simulink model "IEEE33bus_SmartInverter_Hybrid_PSO_English"  (R2026a)
settings: Solver=VariableStepAuto
PreLoadFcn:
  | try, if exist('startup_project','file') == 2, startup_project(); end, catch ME, disp(['PreLoadFcn warning: ' ME.message]); end
InitFcn:
  | try, if exist('ieee33_data','file') == 2, assignin('base','ieee33_visual_network',ieee33_data()); end; if exist('default_control_params','file') == 2, assignin('base','ieee33_visual_control_params',default_control_params()); end; disp('IEEE33 visualization initialized. MATLAB scripts provide numerical results.'); catch ME, disp(['InitFcn warning: ' ME.message]); end
StopFcn:
  | try, disp('IEEE33 visualization stopped. Use main_generate_final_results for refreshed tables and figures.'); catch ME, disp(['StopFcn warning: ' ME.message]); end
settings Model: Creator=ismahin  LastModifiedBy=ismahin

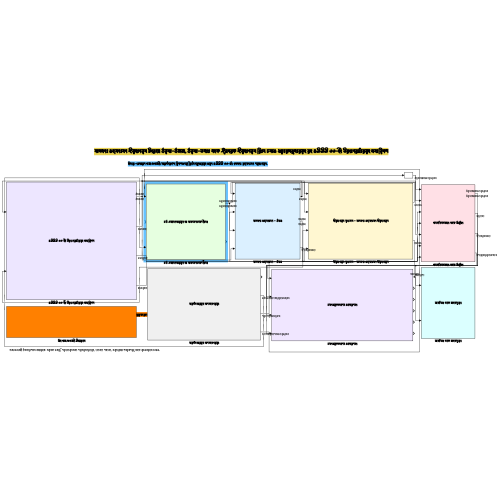
[thumbnail: Simulink's stored preview of the top-level diagram]
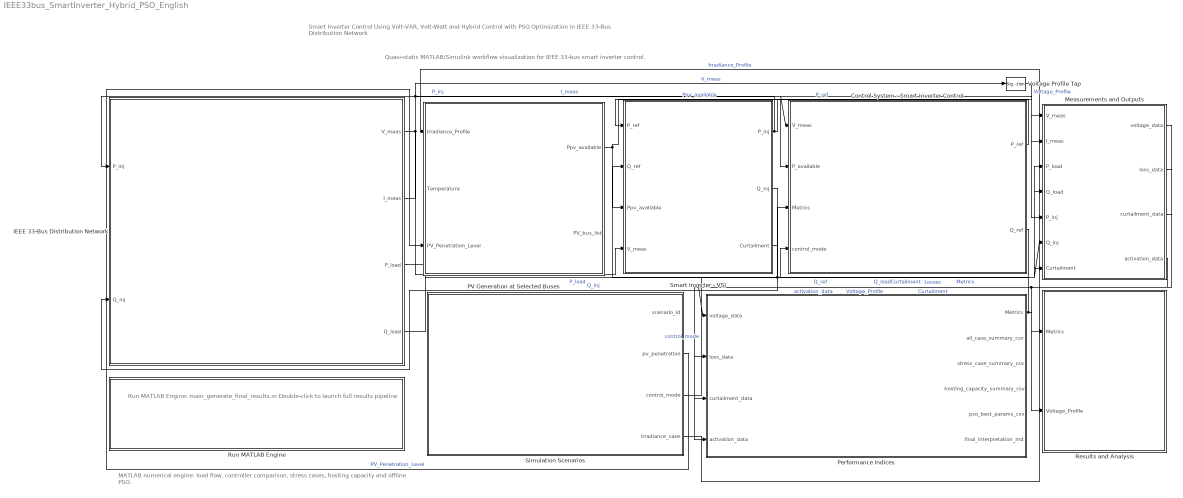
== system IEEE33bus_SmartInverter_Hybrid_PSO_English ==
  note: Run MATLAB Engine:\nmain_generate_final_results.m\nDouble-click to launch full results pipeline
  note: Smart Inverter Control Using Volt-VAR, Volt-Watt and Hybrid Control with PSO Optimization in IEEE 33-Bus Distribution Network
  note: Quasi-static MATLAB/Simulink workflow visualization for IEEE 33-bus smart inverter control.
  note: MATLAB numerical engine: load flow, controller comparison, stress cases, hosting capacity and offline PSO.
  Control System - Smart Inverter Control : Subsystem
      mask Display: color('black'); patch([0 1 1 0],[0 0 1 1],[1.000 0.970 0.820]); disp('Control System - Smart Inverter Control');
  IEEE 33-Bus Distribution Network : Subsystem
      mask Display: color('black'); patch([0 1 1 0],[0 0 1 1],[0.930 0.900 1.000]); disp('IEEE 33-Bus Distribution Network');
  Measurements and Outputs : Subsystem
      mask Display: color('black'); patch([0 1 1 0],[0 0 1 1],[1.000 0.880 0.900]); disp('Measurements and Outputs');
  PV Generation at Selected Buses : Subsystem
      mask Display: color('black'); patch([0 1 1 0],[0 0 1 1],[0.900 1.000 0.880]); disp('PV Generation at Selected Buses');
  Performance Indices : Subsystem
      mask Display: color('black'); patch([0 1 1 0],[0 0 1 1],[0.940 0.900 1.000]); disp('Performance Indices');
  Results and Analysis : Subsystem
      mask Display: color('black'); patch([0 1 1 0],[0 0 1 1],[0.860 1.000 1.000]); disp('Results and Analysis');
  Run MATLAB Engine : Subsystem
      settings: OpenFcn=try, evalin('base','main_generate_final_results'); catch ME, disp(['Pipeline launch failed: ' ME.message]); end
  Simulation Scenarios : Subsystem
      mask Display: color('black'); patch([0 1 1 0],[0 0 1 1],[0.940 0.940 0.940]); disp('Simulation Scenarios');
  Smart Inverter - VSI : Subsystem
      mask Display: color('black'); patch([0 1 1 0],[0 0 1 1],[0.860 0.940 1.000]); disp('Smart Inverter - VSI');
  Voltage Profile Tap : SignalSpecification
  wires:
  Simulation Scenarios/4(irradiance_case) -> PV Generation at Selected Buses/1(Irradiance_Profile)  "Irradiance_Profile"
  Simulation Scenarios/2(pv_penetration) -> PV Generation at Selected Buses/3(PV_Penetration_Level)  "PV_Penetration_Level"
  Simulation Scenarios/3(control_mode) -> Control System - Smart Inverter Control/4(control_mode)  "control_mode"
  PV Generation at Selected Buses/1(Ppv_available) -> Smart Inverter - VSI/3(Ppv_available), Control System - Smart Inverter Control/2(P_available)  "Ppv_available"
  IEEE 33-Bus Distribution Network/1(V_meas) -> Control System - Smart Inverter Control/1(V_meas), Voltage Profile Tap/1, Smart Inverter - VSI/4(V_meas)  "V_meas"
  Control System - Smart Inverter Control/1(P_ref) -> Smart Inverter - VSI/1(P_ref)  "P_ref"
  Control System - Smart Inverter Control/2(Q_ref) -> Smart Inverter - VSI/2(Q_ref)  "Q_ref"
  Smart Inverter - VSI/1(P_inj) -> IEEE 33-Bus Distribution Network/1(P_inj), Measurements and Outputs/5(P_inj)  "P_inj"
  Smart Inverter - VSI/2(Q_inj) -> IEEE 33-Bus Distribution Network/2(Q_inj), Measurements and Outputs/6(Q_inj)  "Q_inj"
  Voltage Profile Tap/1 -> Measurements and Outputs/1(V_meas)  "Voltage_Profile"
  IEEE 33-Bus Distribution Network/2(I_meas) -> Measurements and Outputs/2(I_meas)  "I_meas"
  IEEE 33-Bus Distribution Network/3(P_load) -> Measurements and Outputs/3(P_load)  "P_load"
  IEEE 33-Bus Distribution Network/4(Q_load) -> Measurements and Outputs/4(Q_load)  "Q_load"
  Smart Inverter - VSI/3(Curtailment) -> Measurements and Outputs/7(Curtailment)  "Curtailment"
  Measurements and Outputs/1(voltage_data) -> Performance Indices/1(voltage_data), Results and Analysis/2(Voltage_Profile)  "Voltage_Profile"
  Measurements and Outputs/2(loss_data) -> Performance Indices/2(loss_data)  "Losses"
  Measurements and Outputs/3(curtailment_data) -> Performance Indices/3(curtailment_data)  "Curtailment"
  Measurements and Outputs/4(activation_data) -> Performance Indices/4(activation_data)  "activation_data"
  Performance Indices/1(Metrics) -> Results and Analysis/1(Metrics), Control System - Smart Inverter Control/3(Metrics)  "Metrics"

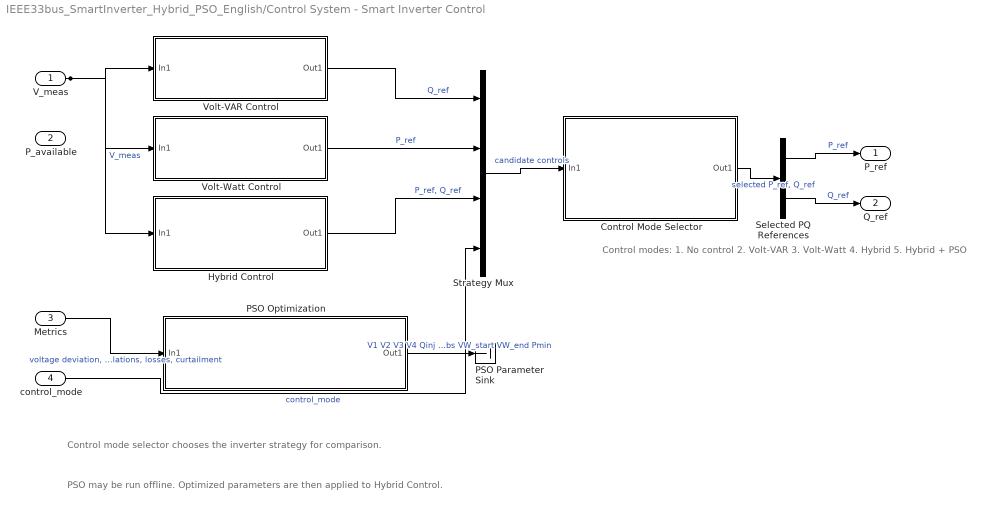
== system IEEE33bus_SmartInverter_Hybrid_PSO_English/Control System - Smart Inverter Control ==
  note: Control modes:\n1. No control\n2. Volt-VAR\n3. Volt-Watt\n4. Hybrid\n5. Hybrid + PSO
  note: Control mode selector chooses the inverter strategy for comparison.
  note: PSO may be run offline. Optimized parameters are then applied to Hybrid Control.
  V_meas : Inport
  P_available : Inport  Port=2
  Metrics : Inport  Port=3
  control_mode : Inport  Port=4
  Control Mode Selector : Subsystem
      mask Display: color('black'); patch([0 1 1 0],[0 0 1 1],[1.000 0.950 0.780]); disp('Control Mode Selector');
  Hybrid Control : Subsystem
      mask Display: color('black'); patch([0 1 1 0],[0 0 1 1],[1.000 0.900 0.580]); disp('Hybrid: Volt-VAR + Volt-Watt');
  PSO Optimization : Subsystem
      mask Display: color('black'); patch([0 1 1 0],[0 0 1 1],[1.000 0.780 0.900]); disp('PSO Optimization (Offline)');
  PSO Parameter Sink : Terminator
  Selected PQ References : Demux  Outputs=2
  Strategy Mux : Mux
  Volt-VAR Control : Subsystem
      mask Display: color('black'); patch([0 1 1 0],[0 0 1 1],[1.000 0.930 0.660]); disp('Volt-VAR Control  Q = f(V)');
  Volt-Watt Control : Subsystem
      mask Display: color('black'); patch([0 1 1 0],[0 0 1 1],[1.000 0.930 0.660]); disp('Volt-Watt Control  P = f(V)');
  P_ref : Outport
  Q_ref : Outport  Port=2
  wires:
  V_meas/1 -> Volt-VAR Control/1(In1), Volt-Watt Control/1(In1), Hybrid Control/1(In1)  "V_meas"
  Metrics/1 -> PSO Optimization/1(In1)  "voltage deviation, violations, losses, curtailment"
  Volt-VAR Control/1(Out1) -> Strategy Mux/1  "Q_ref"
  Volt-Watt Control/1(Out1) -> Strategy Mux/2  "P_ref"
  Hybrid Control/1(Out1) -> Strategy Mux/3  "P_ref, Q_ref"
  control_mode/1 -> Strategy Mux/4  "control_mode"
  Strategy Mux/1 -> Control Mode Selector/1(In1)  "candidate controls"
  Control Mode Selector/1(Out1) -> Selected PQ References/1  "selected P_ref, Q_ref"
  Selected PQ References/1 -> P_ref/1  "P_ref"
  Selected PQ References/2 -> Q_ref/1  "Q_ref"
  PSO Optimization/1(Out1) -> PSO Parameter Sink/1  "V1 V2 V3 V4 Qinj Qabs VW_start VW_end Pmin"

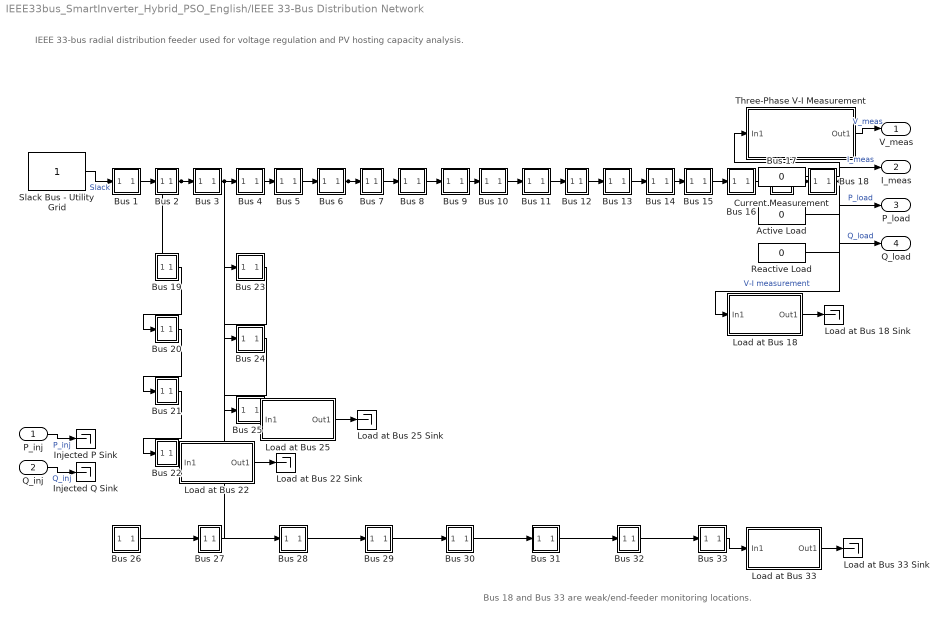
== system IEEE33bus_SmartInverter_Hybrid_PSO_English/IEEE 33-Bus Distribution Network ==
  note: IEEE 33-bus radial distribution feeder used for voltage regulation and PV hosting capacity analysis.
  note: Bus 18 and Bus 33 are weak/end-feeder monitoring locations.
  P_inj : Inport
  Q_inj : Inport  Port=2
  Active Load : Constant  Value=0
  Bus 1 : Subsystem
      mask Display: color('black'); patch([0 1 1 0],[0 0 1 1],[0.820 0.820 0.820]); disp('1');
  Bus 10 : Subsystem
      mask Display: color('black'); patch([0 1 1 0],[0 0 1 1],[0.820 0.820 0.820]); disp('10');
  Bus 11 : Subsystem
      mask Display: color('black'); patch([0 1 1 0],[0 0 1 1],[0.820 0.820 0.820]); disp('11');
  Bus 12 : Subsystem
      mask Display: color('black'); patch([0 1 1 0],[0 0 1 1],[0.820 0.820 0.820]); disp('12');
  Bus 13 : Subsystem
      mask Display: color('black'); patch([0 1 1 0],[0 0 1 1],[0.820 0.820 0.820]); disp('13');
  Bus 14 : Subsystem
      mask Display: color('black'); patch([0 1 1 0],[0 0 1 1],[0.820 0.820 0.820]); disp('14');
  Bus 15 : Subsystem
      mask Display: color('black'); patch([0 1 1 0],[0 0 1 1],[0.820 0.820 0.820]); disp('15');
  Bus 16 : Subsystem
      mask Display: color('black'); patch([0 1 1 0],[0 0 1 1],[0.820 0.820 0.820]); disp('16');
  Bus 17 : Subsystem
      mask Display: color('black'); patch([0 1 1 0],[0 0 1 1],[0.820 0.820 0.820]); disp('17');
  Bus 18 : Subsystem
      mask Display: color('black'); patch([0 1 1 0],[0 0 1 1],[0.820 0.820 0.820]); disp('18');
  Bus 19 : Subsystem
      mask Display: color('black'); patch([0 1 1 0],[0 0 1 1],[0.820 0.820 0.820]); disp('19');
  Bus 2 : Subsystem
      mask Display: color('black'); patch([0 1 1 0],[0 0 1 1],[0.820 0.820 0.820]); disp('2');
  Bus 20 : Subsystem
      mask Display: color('black'); patch([0 1 1 0],[0 0 1 1],[0.820 0.820 0.820]); disp('20');
  Bus 21 : Subsystem
      mask Display: color('black'); patch([0 1 1 0],[0 0 1 1],[0.820 0.820 0.820]); disp('21');
  Bus 22 : Subsystem
      mask Display: color('black'); patch([0 1 1 0],[0 0 1 1],[0.820 0.820 0.820]); disp('22');
  Bus 23 : Subsystem
      mask Display: color('black'); patch([0 1 1 0],[0 0 1 1],[0.820 0.820 0.820]); disp('23');
  Bus 24 : Subsystem
      mask Display: color('black'); patch([0 1 1 0],[0 0 1 1],[0.820 0.820 0.820]); disp('24');
  Bus 25 : Subsystem
      mask Display: color('black'); patch([0 1 1 0],[0 0 1 1],[0.820 0.820 0.820]); disp('25');
  Bus 26 : Subsystem
      mask Display: color('black'); patch([0 1 1 0],[0 0 1 1],[0.820 0.820 0.820]); disp('26');
  Bus 27 : Subsystem
      mask Display: color('black'); patch([0 1 1 0],[0 0 1 1],[0.820 0.820 0.820]); disp('27');
  Bus 28 : Subsystem
      mask Display: color('black'); patch([0 1 1 0],[0 0 1 1],[0.820 0.820 0.820]); disp('28');
  Bus 29 : Subsystem
      mask Display: color('black'); patch([0 1 1 0],[0 0 1 1],[0.820 0.820 0.820]); disp('29');
  Bus 3 : Subsystem
      mask Display: color('black'); patch([0 1 1 0],[0 0 1 1],[0.820 0.820 0.820]); disp('3');
  Bus 30 : Subsystem
      mask Display: color('black'); patch([0 1 1 0],[0 0 1 1],[0.820 0.820 0.820]); disp('30');
  Bus 31 : Subsystem
      mask Display: color('black'); patch([0 1 1 0],[0 0 1 1],[0.820 0.820 0.820]); disp('31');
  Bus 32 : Subsystem
      mask Display: color('black'); patch([0 1 1 0],[0 0 1 1],[0.820 0.820 0.820]); disp('32');
  Bus 33 : Subsystem
      mask Display: color('black'); patch([0 1 1 0],[0 0 1 1],[0.820 0.820 0.820]); disp('33');
  Bus 4 : Subsystem
      mask Display: color('black'); patch([0 1 1 0],[0 0 1 1],[0.820 0.820 0.820]); disp('4');
  Bus 5 : Subsystem
      mask Display: color('black'); patch([0 1 1 0],[0 0 1 1],[0.820 0.820 0.820]); disp('5');
  Bus 6 : Subsystem
      mask Display: color('black'); patch([0 1 1 0],[0 0 1 1],[0.820 0.820 0.820]); disp('6');
  Bus 7 : Subsystem
      mask Display: color('black'); patch([0 1 1 0],[0 0 1 1],[0.820 0.820 0.820]); disp('7');
  Bus 8 : Subsystem
      mask Display: color('black'); patch([0 1 1 0],[0 0 1 1],[0.820 0.820 0.820]); disp('8');
  Bus 9 : Subsystem
      mask Display: color('black'); patch([0 1 1 0],[0 0 1 1],[0.820 0.820 0.820]); disp('9');
  Current Measurement : Constant  Value=0
  Injected P Sink : Terminator
  Injected Q Sink : Terminator
  Load at Bus 18 : Subsystem
      mask Display: color('black'); patch([0 1 1 0],[0 0 1 1],[1.000 0.880 0.820]); disp('Load\nBus 18');
  Load at Bus 18 Sink : Terminator
  Load at Bus 22 : Subsystem
      mask Display: color('black'); patch([0 1 1 0],[0 0 1 1],[1.000 0.880 0.820]); disp('Load\nBus 22');
  Load at Bus 22 Sink : Terminator
  Load at Bus 25 : Subsystem
      mask Display: color('black'); patch([0 1 1 0],[0 0 1 1],[1.000 0.880 0.820]); disp('Load\nBus 25');
  Load at Bus 25 Sink : Terminator
  Load at Bus 33 : Subsystem
      mask Display: color('black'); patch([0 1 1 0],[0 0 1 1],[1.000 0.880 0.820]); disp('Load\nBus 33');
  Load at Bus 33 Sink : Terminator
  Reactive Load : Constant  Value=0
  Slack Bus - Utility Grid : Constant
  Three-Phase V-I Measurement : Subsystem
      mask Display: color('black'); patch([0 1 1 0],[0 0 1 1],[1.000 0.940 0.800]); disp('Three-Phase V-I Measurement');
  V_meas : Outport
  I_meas : Outport  Port=2
  P_load : Outport  Port=3
  Q_load : Outport  Port=4
  wires:
  Slack Bus - Utility Grid/1 -> Bus 1/1(In1)  "Slack"
  Bus 1/1(Out1) -> Bus 2/1(In1)
  Bus 2/1(Out1) -> Bus 3/1(In1), Bus 19/1(In1)
  Bus 3/1(Out1) -> Bus 4/1(In1), Bus 23/1(In1)
  Bus 4/1(Out1) -> Bus 5/1(In1)
  Bus 5/1(Out1) -> Bus 6/1(In1)
  Bus 6/1(Out1) -> Bus 7/1(In1), Bus 26/1(In1)
  Bus 7/1(Out1) -> Bus 8/1(In1)
  Bus 8/1(Out1) -> Bus 9/1(In1)
  Bus 9/1(Out1) -> Bus 10/1(In1)
  Bus 10/1(Out1) -> Bus 11/1(In1)
  Bus 11/1(Out1) -> Bus 12/1(In1)
  Bus 12/1(Out1) -> Bus 13/1(In1)
  Bus 13/1(Out1) -> Bus 14/1(In1)
  Bus 14/1(Out1) -> Bus 15/1(In1)
  Bus 15/1(Out1) -> Bus 16/1(In1)
  Bus 16/1(Out1) -> Bus 17/1(In1)
  Bus 17/1(Out1) -> Bus 18/1(In1)
  Bus 19/1(Out1) -> Bus 20/1(In1)
  Bus 20/1(Out1) -> Bus 21/1(In1)
  Bus 21/1(Out1) -> Bus 22/1(In1)
  Bus 23/1(Out1) -> Bus 24/1(In1)
  Bus 24/1(Out1) -> Bus 25/1(In1)
  Bus 26/1(Out1) -> Bus 27/1(In1)
  Bus 27/1(Out1) -> Bus 28/1(In1)
  Bus 28/1(Out1) -> Bus 29/1(In1)
  Bus 29/1(Out1) -> Bus 30/1(In1)
  Bus 30/1(Out1) -> Bus 31/1(In1)
  Bus 31/1(Out1) -> Bus 32/1(In1)
  Bus 32/1(Out1) -> Bus 33/1(In1)
  Bus 18/1(Out1) -> Three-Phase V-I Measurement/1(In1), Load at Bus 18/1(In1)  "V-I measurement"
  Three-Phase V-I Measurement/1(Out1) -> V_meas/1  "V_meas"
  Current Measurement/1 -> I_meas/1  "I_meas"
  Active Load/1 -> P_load/1  "P_load"
  Reactive Load/1 -> Q_load/1  "Q_load"
  Load at Bus 18/1(Out1) -> Load at Bus 18 Sink/1
  Bus 22/1(Out1) -> Load at Bus 22/1(In1)
  Load at Bus 22/1(Out1) -> Load at Bus 22 Sink/1
  Bus 25/1(Out1) -> Load at Bus 25/1(In1)
  Load at Bus 25/1(Out1) -> Load at Bus 25 Sink/1
  Bus 33/1(Out1) -> Load at Bus 33/1(In1)
  Load at Bus 33/1(Out1) -> Load at Bus 33 Sink/1
  P_inj/1 -> Injected P Sink/1  "P_inj"
  Q_inj/1 -> Injected Q Sink/1  "Q_inj"

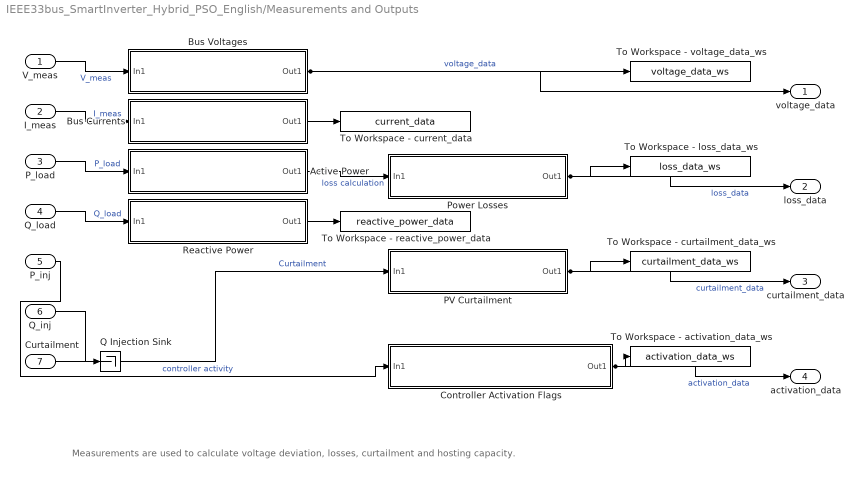
== system IEEE33bus_SmartInverter_Hybrid_PSO_English/Measurements and Outputs ==
  note: Measurements are used to calculate voltage deviation, losses, curtailment and hosting capacity.
  V_meas : Inport
  I_meas : Inport  Port=2
  P_load : Inport  Port=3
  Q_load : Inport  Port=4
  P_inj : Inport  Port=5
  Q_inj : Inport  Port=6
  Curtailment : Inport  Port=7
  Active Power : Subsystem
      mask Display: color('black'); patch([0 1 1 0],[0 0 1 1],[1.000 0.920 0.920]); disp('Active Power (kW)');
  Bus Currents : Subsystem
      mask Display: color('black'); patch([0 1 1 0],[0 0 1 1],[1.000 0.920 0.920]); disp('Bus Currents (A)');
  Bus Voltages : Subsystem
      mask Display: color('black'); patch([0 1 1 0],[0 0 1 1],[1.000 0.920 0.920]); disp('Bus Voltages (p.u.)');
  Controller Activation Flags : Subsystem
      mask Display: color('black'); patch([0 1 1 0],[0 0 1 1],[1.000 0.860 0.880]); disp('Controller Activation Flags');
  PV Curtailment : Subsystem
      mask Display: color('black'); patch([0 1 1 0],[0 0 1 1],[1.000 0.860 0.880]); disp('PV Curtailment (kWh)');
  Power Losses : Subsystem
      mask Display: color('black'); patch([0 1 1 0],[0 0 1 1],[1.000 0.860 0.880]); disp('Power Losses (kW)');
  Q Injection Sink : Terminator
  Reactive Power : Subsystem
      mask Display: color('black'); patch([0 1 1 0],[0 0 1 1],[1.000 0.920 0.920]); disp('Reactive Power (kVAr)');
  To Workspace - activation_data_ws : ToWorkspace  VariableName=activation_data_ws  SampleTime=-1
  To Workspace - current_data : ToWorkspace  VariableName=current_data  SampleTime=-1
  To Workspace - curtailment_data_ws : ToWorkspace  VariableName=curtailment_data_ws  SampleTime=-1
  To Workspace - loss_data_ws : ToWorkspace  VariableName=loss_data_ws  SampleTime=-1
  To Workspace - reactive_power_data : ToWorkspace  VariableName=reactive_power_data  SampleTime=-1
  To Workspace - voltage_data_ws : ToWorkspace  VariableName=voltage_data_ws  SampleTime=-1
  voltage_data : Outport
  loss_data : Outport  Port=2
  curtailment_data : Outport  Port=3
  activation_data : Outport  Port=4
  wires:
  V_meas/1 -> Bus Voltages/1(In1)  "V_meas"
  Bus Voltages/1(Out1) -> voltage_data/1, To Workspace - voltage_data_ws/1  "voltage_data"
  I_meas/1 -> Bus Currents/1(In1)  "I_meas"
  P_load/1 -> Active Power/1(In1)  "P_load"
  Q_load/1 -> Reactive Power/1(In1)  "Q_load"
  Active Power/1(Out1) -> Power Losses/1(In1)  "loss calculation"
  Power Losses/1(Out1) -> loss_data/1, To Workspace - loss_data_ws/1  "loss_data"
  Curtailment/1 -> PV Curtailment/1(In1)  "Curtailment"
  PV Curtailment/1(Out1) -> curtailment_data/1, To Workspace - curtailment_data_ws/1  "curtailment_data"
  P_inj/1 -> Controller Activation Flags/1(In1)  "controller activity"
  Controller Activation Flags/1(Out1) -> activation_data/1, To Workspace - activation_data_ws/1  "activation_data"
  Bus Currents/1(Out1) -> To Workspace - current_data/1
  Reactive Power/1(Out1) -> To Workspace - reactive_power_data/1
  Q_inj/1 -> Q Injection Sink/1

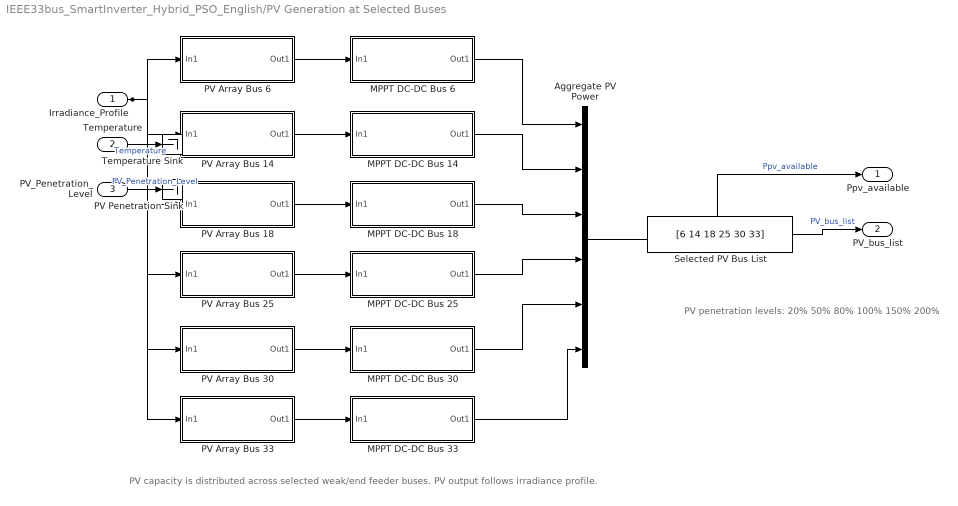
== system IEEE33bus_SmartInverter_Hybrid_PSO_English/PV Generation at Selected Buses ==
  note: PV penetration levels:\n20%\n50%\n80%\n100%\n150%\n200%
  note: PV capacity is distributed across selected weak/end feeder buses. PV output follows irradiance profile.
  Irradiance_Profile : Inport
  Temperature : Inport  Port=2
  PV_Penetration_Level : Inport  Port=3
  Aggregate PV Power : Mux  Inputs=6
  MPPT DC-DC Bus 14 : Subsystem
      mask Display: color('black'); patch([0 1 1 0],[0 0 1 1],[0.860 0.980 0.820]); disp('DC-DC / MPPT');
  MPPT DC-DC Bus 18 : Subsystem
      mask Display: color('black'); patch([0 1 1 0],[0 0 1 1],[0.860 0.980 0.820]); disp('DC-DC / MPPT');
  MPPT DC-DC Bus 25 : Subsystem
      mask Display: color('black'); patch([0 1 1 0],[0 0 1 1],[0.860 0.980 0.820]); disp('DC-DC / MPPT');
  MPPT DC-DC Bus 30 : Subsystem
      mask Display: color('black'); patch([0 1 1 0],[0 0 1 1],[0.860 0.980 0.820]); disp('DC-DC / MPPT');
  MPPT DC-DC Bus 33 : Subsystem
      mask Display: color('black'); patch([0 1 1 0],[0 0 1 1],[0.860 0.980 0.820]); disp('DC-DC / MPPT');
  MPPT DC-DC Bus 6 : Subsystem
      mask Display: color('black'); patch([0 1 1 0],[0 0 1 1],[0.860 0.980 0.820]); disp('DC-DC / MPPT');
  PV Array Bus 14 : Subsystem
      mask Display: color('black'); patch([0 1 1 0],[0 0 1 1],[0.720 0.940 0.720]); disp('PV Array\nBus 14');
  PV Array Bus 18 : Subsystem
      mask Display: color('black'); patch([0 1 1 0],[0 0 1 1],[0.720 0.940 0.720]); disp('PV Array\nBus 18');
  PV Array Bus 25 : Subsystem
      mask Display: color('black'); patch([0 1 1 0],[0 0 1 1],[0.720 0.940 0.720]); disp('PV Array\nBus 25');
  PV Array Bus 30 : Subsystem
      mask Display: color('black'); patch([0 1 1 0],[0 0 1 1],[0.720 0.940 0.720]); disp('PV Array\nBus 30');
  PV Array Bus 33 : Subsystem
      mask Display: color('black'); patch([0 1 1 0],[0 0 1 1],[0.720 0.940 0.720]); disp('PV Array\nBus 33');
  PV Array Bus 6 : Subsystem
      mask Display: color('black'); patch([0 1 1 0],[0 0 1 1],[0.720 0.940 0.720]); disp('PV Array\nBus 6');
  PV Penetration Sink : Terminator
  Selected PV Bus List : Constant  Value=[6 14 18 25 30 33]
  Temperature Sink : Terminator
  Ppv_available : Outport
  PV_bus_list : Outport  Port=2
  wires:
  Irradiance_Profile/1 -> PV Array Bus 6/1(In1), PV Array Bus 14/1(In1), PV Array Bus 18/1(In1), PV Array Bus 25/1(In1), PV Array Bus 30/1(In1), PV Array Bus 33/1(In1)
  PV Array Bus 6/1(Out1) -> MPPT DC-DC Bus 6/1(In1)
  PV Array Bus 14/1(Out1) -> MPPT DC-DC Bus 14/1(In1)
  PV Array Bus 18/1(Out1) -> MPPT DC-DC Bus 18/1(In1)
  PV Array Bus 25/1(Out1) -> MPPT DC-DC Bus 25/1(In1)
  PV Array Bus 30/1(Out1) -> MPPT DC-DC Bus 30/1(In1)
  PV Array Bus 33/1(Out1) -> MPPT DC-DC Bus 33/1(In1)
  MPPT DC-DC Bus 6/1(Out1) -> Aggregate PV Power/1
  MPPT DC-DC Bus 14/1(Out1) -> Aggregate PV Power/2
  MPPT DC-DC Bus 18/1(Out1) -> Aggregate PV Power/3
  MPPT DC-DC Bus 25/1(Out1) -> Aggregate PV Power/4
  MPPT DC-DC Bus 30/1(Out1) -> Aggregate PV Power/5
  MPPT DC-DC Bus 33/1(Out1) -> Aggregate PV Power/6
  Aggregate PV Power/1 -> Ppv_available/1  "Ppv_available"
  Selected PV Bus List/1 -> PV_bus_list/1  "PV_bus_list"
  Temperature/1 -> Temperature Sink/1  "Temperature"
  PV_Penetration_Level/1 -> PV Penetration Sink/1  "PV_Penetration_Level"

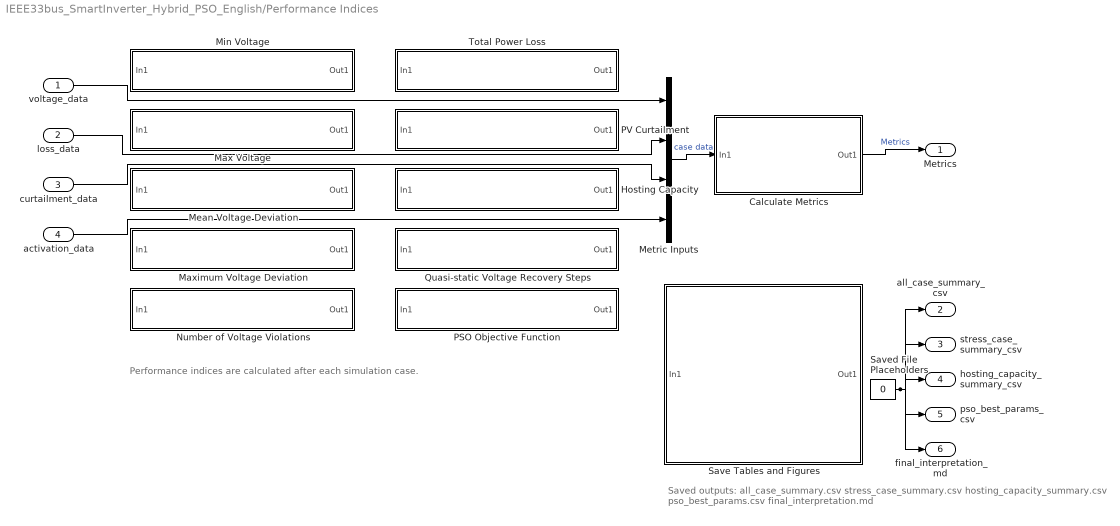
== system IEEE33bus_SmartInverter_Hybrid_PSO_English/Performance Indices ==
  note: Saved outputs:\nall_case_summary.csv\nstress_case_summary.csv\nhosting_capacity_summary.csv\npso_best_params.csv\nfinal_interpretation.md
  note: Performance indices are calculated after each simulation case.
  voltage_data : Inport
  loss_data : Inport  Port=2
  curtailment_data : Inport  Port=3
  activation_data : Inport  Port=4
  Calculate Metrics : Subsystem
      mask Display: color('black'); patch([0 1 1 0],[0 0 1 1],[0.880 0.820 1.000]); disp('Calculate Metrics');
  Hosting Capacity : Subsystem
      mask Display: color('black'); patch([0 1 1 0],[0 0 1 1],[0.960 0.930 1.000]); disp('Hosting Capacity');
  Max Voltage : Subsystem
      mask Display: color('black'); patch([0 1 1 0],[0 0 1 1],[0.960 0.930 1.000]); disp('Max Voltage');
  Maximum Voltage Deviation : Subsystem
      mask Display: color('black'); patch([0 1 1 0],[0 0 1 1],[0.960 0.930 1.000]); disp('Maximum Voltage Deviation');
  Mean Voltage Deviation : Subsystem
      mask Display: color('black'); patch([0 1 1 0],[0 0 1 1],[0.960 0.930 1.000]); disp('Mean Voltage Deviation');
  Metric Inputs : Mux
  Min Voltage : Subsystem
      mask Display: color('black'); patch([0 1 1 0],[0 0 1 1],[0.960 0.930 1.000]); disp('Min Voltage');
  Number of Voltage Violations : Subsystem
      mask Display: color('black'); patch([0 1 1 0],[0 0 1 1],[0.960 0.930 1.000]); disp('Number of Voltage Violations');
  PSO Objective Function : Subsystem
      mask Display: color('black'); patch([0 1 1 0],[0 0 1 1],[0.960 0.930 1.000]); disp('PSO Objective Function');
  PV Curtailment : Subsystem
      mask Display: color('black'); patch([0 1 1 0],[0 0 1 1],[0.960 0.930 1.000]); disp('PV Curtailment');
  Quasi-static Voltage Recovery Steps : Subsystem
      mask Display: color('black'); patch([0 1 1 0],[0 0 1 1],[0.960 0.930 1.000]); disp('Quasi-static Voltage Recovery Steps');
  Save Tables and Figures : Subsystem
      mask Display: color('black'); patch([0 1 1 0],[0 0 1 1],[0.900 0.840 1.000]); disp('Save Tables and Figures');
  Saved File Placeholders : Constant  Value=0
  Total Power Loss : Subsystem
      mask Display: color('black'); patch([0 1 1 0],[0 0 1 1],[0.960 0.930 1.000]); disp('Total Power Loss');
  Metrics : Outport
  all_case_summary_csv : Outport  Port=2
  stress_case_summary_csv : Outport  Port=3
  hosting_capacity_summary_csv : Outport  Port=4
  pso_best_params_csv : Outport  Port=5
  final_interpretation_md : Outport  Port=6
  wires:
  voltage_data/1 -> Metric Inputs/1
  loss_data/1 -> Metric Inputs/2
  curtailment_data/1 -> Metric Inputs/3
  activation_data/1 -> Metric Inputs/4
  Metric Inputs/1 -> Calculate Metrics/1(In1)  "case data"
  Calculate Metrics/1(Out1) -> Metrics/1  "Metrics"
  Saved File Placeholders/1 -> all_case_summary_csv/1, stress_case_summary_csv/1, hosting_capacity_summary_csv/1, pso_best_params_csv/1, final_interpretation_md/1

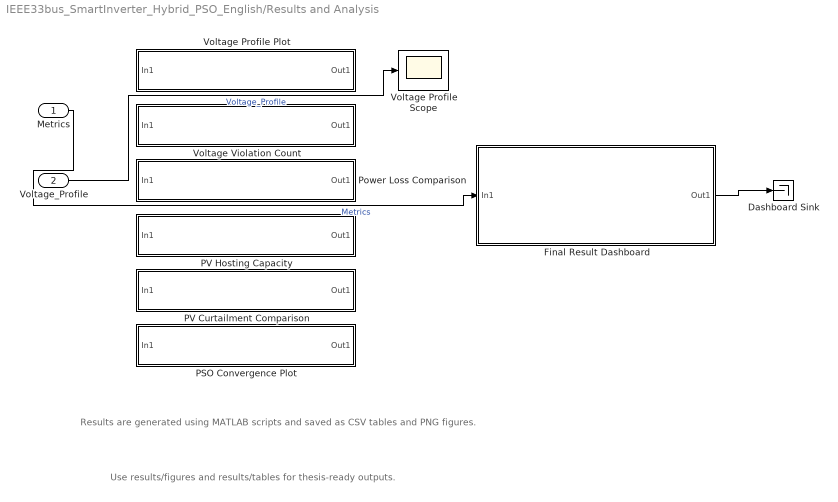
== system IEEE33bus_SmartInverter_Hybrid_PSO_English/Results and Analysis ==
  note: Results are generated using MATLAB scripts and saved as CSV tables and PNG figures.
  note: Use results/figures and results/tables for thesis-ready outputs.
  Metrics : Inport
  Voltage_Profile : Inport  Port=2
  Dashboard Sink : Terminator
  Final Result Dashboard : Subsystem
      mask Display: color('black'); patch([0 1 1 0],[0 0 1 1],[0.720 0.960 1.000]); disp('Final Result Dashboard');
  PSO Convergence Plot : Subsystem
      mask Display: color('black'); patch([0 1 1 0],[0 0 1 1],[0.840 0.980 1.000]); disp('PSO Convergence Plot');
  PV Curtailment Comparison : Subsystem
      mask Display: color('black'); patch([0 1 1 0],[0 0 1 1],[0.840 0.980 1.000]); disp('PV Curtailment Comparison');
  PV Hosting Capacity : Subsystem
      mask Display: color('black'); patch([0 1 1 0],[0 0 1 1],[0.840 0.980 1.000]); disp('PV Hosting Capacity');
  Power Loss Comparison : Subsystem
      mask Display: color('black'); patch([0 1 1 0],[0 0 1 1],[0.840 0.980 1.000]); disp('Power Loss Comparison');
  Voltage Profile Plot : Subsystem
      mask Display: color('black'); patch([0 1 1 0],[0 0 1 1],[0.840 0.980 1.000]); disp('Voltage Profile Plot');
  Voltage Profile Scope : Scope
  Voltage Violation Count : Subsystem
      mask Display: color('black'); patch([0 1 1 0],[0 0 1 1],[0.840 0.980 1.000]); disp('Voltage Violation Count');
  wires:
  Voltage_Profile/1 -> Voltage Profile Scope/1  "Voltage_Profile"
  Metrics/1 -> Final Result Dashboard/1(In1)  "Metrics"
  Final Result Dashboard/1(Out1) -> Dashboard Sink/1

== system IEEE33bus_SmartInverter_Hybrid_PSO_English/Run MATLAB Engine ==

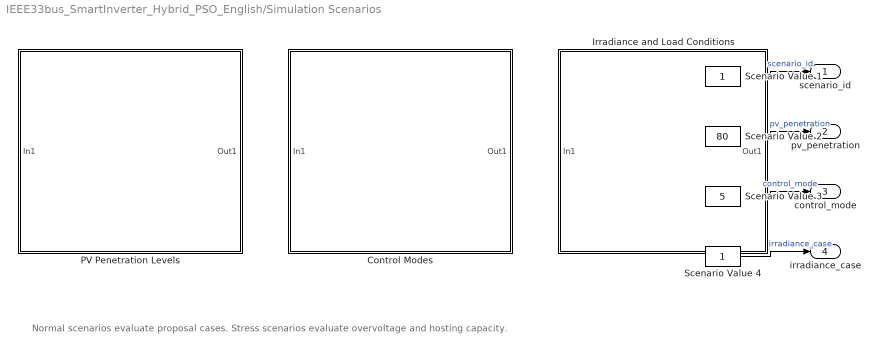
== system IEEE33bus_SmartInverter_Hybrid_PSO_English/Simulation Scenarios ==
  note: Normal scenarios evaluate proposal cases. Stress scenarios evaluate overvoltage and hosting capacity.
  Control Modes : Subsystem
      mask Display: color('black'); patch([0 1 1 0],[0 0 1 1],[0.980 0.980 0.980]); disp('Control Modes\nNo control\nVolt-VAR\nVolt-Watt\nHybrid\nHybrid + PSO');
  Irradiance and Load Conditions : Subsystem
      mask Display: color('black'); patch([0 1 1 0],[0 0 1 1],[0.980 0.980 0.980]); disp('Irradiance / Load\nClear sky\nPartial cloud\nLow irradiance\nStress: low load, high PV');
  PV Penetration Levels : Subsystem
      mask Display: color('black'); patch([0 1 1 0],[0 0 1 1],[0.980 0.980 0.980]); disp('PV Penetration Levels\n20%  50%  80%\n100%  150%  200%');
  Scenario Value 1 : Constant
  Scenario Value 2 : Constant  Value=80
  Scenario Value 3 : Constant  Value=5
  Scenario Value 4 : Constant
  scenario_id : Outport
  pv_penetration : Outport  Port=2
  control_mode : Outport  Port=3
  irradiance_case : Outport  Port=4
  wires:
  Scenario Value 1/1 -> scenario_id/1  "scenario_id"
  Scenario Value 2/1 -> pv_penetration/1  "pv_penetration"
  Scenario Value 3/1 -> control_mode/1  "control_mode"
  Scenario Value 4/1 -> irradiance_case/1  "irradiance_case"

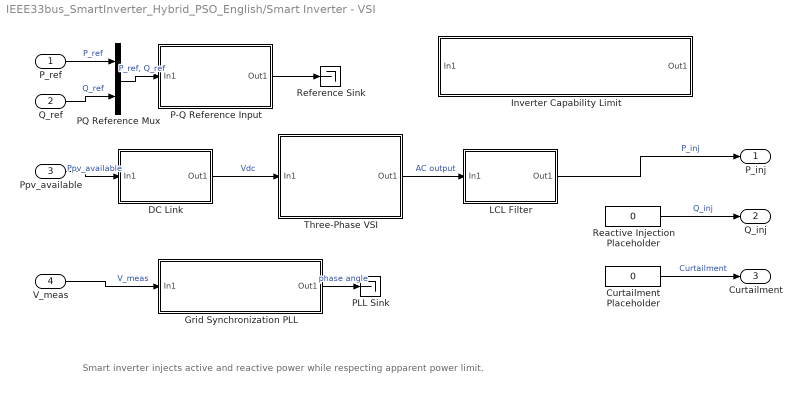
== system IEEE33bus_SmartInverter_Hybrid_PSO_English/Smart Inverter - VSI ==
  note: Smart inverter injects active and reactive power while respecting apparent power limit.
  P_ref : Inport
  Q_ref : Inport  Port=2
  Ppv_available : Inport  Port=3
  V_meas : Inport  Port=4
  Curtailment Placeholder : Constant  Value=0
  DC Link : Subsystem
      mask Display: color('black'); patch([0 1 1 0],[0 0 1 1],[0.780 0.910 1.000]); disp('DC Link');
  Grid Synchronization PLL : Subsystem
      mask Display: color('black'); patch([0 1 1 0],[0 0 1 1],[0.880 0.950 1.000]); disp('Grid Synchronization / PLL');
  Inverter Capability Limit : Subsystem
      mask Display: color('black'); patch([0 1 1 0],[0 0 1 1],[1.000 0.940 0.800]); disp('Capability Limit: sqrt(P^2 + Q^2) <= S_inv');
  LCL Filter : Subsystem
      mask Display: color('black'); patch([0 1 1 0],[0 0 1 1],[0.820 0.930 1.000]); disp('LCL Filter');
  P-Q Reference Input : Subsystem
      mask Display: color('black'); patch([0 1 1 0],[0 0 1 1],[1.000 0.960 0.780]); disp('P/Q Reference Input');
  PLL Sink : Terminator
  PQ Reference Mux : Mux  Inputs=2
  Reactive Injection Placeholder : Constant  Value=0
  Reference Sink : Terminator
  Three-Phase VSI : Subsystem
      mask Display: color('black'); patch([0 1 1 0],[0 0 1 1],[0.720 0.880 1.000]); disp('Three-Phase VSI');
  P_inj : Outport
  Q_inj : Outport  Port=2
  Curtailment : Outport  Port=3
  wires:
  Ppv_available/1 -> DC Link/1(In1)  "Ppv_available"
  DC Link/1(Out1) -> Three-Phase VSI/1(In1)  "Vdc"
  Three-Phase VSI/1(Out1) -> LCL Filter/1(In1)  "AC output"
  LCL Filter/1(Out1) -> P_inj/1  "P_inj"
  P_ref/1 -> PQ Reference Mux/1  "P_ref"
  Q_ref/1 -> PQ Reference Mux/2  "Q_ref"
  PQ Reference Mux/1 -> P-Q Reference Input/1(In1)  "P_ref, Q_ref"
  P-Q Reference Input/1(Out1) -> Reference Sink/1
  V_meas/1 -> Grid Synchronization PLL/1(In1)  "V_meas"
  Grid Synchronization PLL/1(Out1) -> PLL Sink/1  "phase angle"
  Reactive Injection Placeholder/1 -> Q_inj/1  "Q_inj"
  Curtailment Placeholder/1 -> Curtailment/1  "Curtailment"

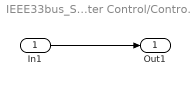
== system IEEE33bus_SmartInverter_Hybrid_PSO_English/Control System - Smart Inverter Control/Control Mode Selector ==
  In1 : Inport
  Out1 : Outport
  wires:
  In1/1 -> Out1/1

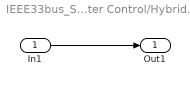
== system IEEE33bus_SmartInverter_Hybrid_PSO_English/Control System - Smart Inverter Control/Hybrid Control ==
  In1 : Inport
  Out1 : Outport
  wires:
  In1/1 -> Out1/1

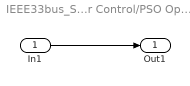
== system IEEE33bus_SmartInverter_Hybrid_PSO_English/Control System - Smart Inverter Control/PSO Optimization ==
  In1 : Inport
  Out1 : Outport
  wires:
  In1/1 -> Out1/1

== system IEEE33bus_SmartInverter_Hybrid_PSO_English/Control System - Smart Inverter Control/Volt-VAR Control ==
  In1 : Inport
  Out1 : Outport
  wires:
  In1/1 -> Out1/1

== system IEEE33bus_SmartInverter_Hybrid_PSO_English/Control System - Smart Inverter Control/Volt-Watt Control ==
  In1 : Inport
  Out1 : Outport
  wires:
  In1/1 -> Out1/1

== system IEEE33bus_SmartInverter_Hybrid_PSO_English/IEEE 33-Bus Distribution Network/Bus 1 ==
  In1 : Inport
  Out1 : Outport
  wires:
  In1/1 -> Out1/1

== system IEEE33bus_SmartInverter_Hybrid_PSO_English/IEEE 33-Bus Distribution Network/Bus 10 ==
  In1 : Inport
  Out1 : Outport
  wires:
  In1/1 -> Out1/1

== system IEEE33bus_SmartInverter_Hybrid_PSO_English/IEEE 33-Bus Distribution Network/Bus 11 ==
  In1 : Inport
  Out1 : Outport
  wires:
  In1/1 -> Out1/1

== system IEEE33bus_SmartInverter_Hybrid_PSO_English/IEEE 33-Bus Distribution Network/Bus 12 ==
  In1 : Inport
  Out1 : Outport
  wires:
  In1/1 -> Out1/1

== system IEEE33bus_SmartInverter_Hybrid_PSO_English/IEEE 33-Bus Distribution Network/Bus 13 ==
  In1 : Inport
  Out1 : Outport
  wires:
  In1/1 -> Out1/1

== system IEEE33bus_SmartInverter_Hybrid_PSO_English/IEEE 33-Bus Distribution Network/Bus 14 ==
  In1 : Inport
  Out1 : Outport
  wires:
  In1/1 -> Out1/1

== system IEEE33bus_SmartInverter_Hybrid_PSO_English/IEEE 33-Bus Distribution Network/Bus 15 ==
  In1 : Inport
  Out1 : Outport
  wires:
  In1/1 -> Out1/1

== system IEEE33bus_SmartInverter_Hybrid_PSO_English/IEEE 33-Bus Distribution Network/Bus 16 ==
  In1 : Inport
  Out1 : Outport
  wires:
  In1/1 -> Out1/1

== system IEEE33bus_SmartInverter_Hybrid_PSO_English/IEEE 33-Bus Distribution Network/Bus 17 ==
  In1 : Inport
  Out1 : Outport
  wires:
  In1/1 -> Out1/1

== system IEEE33bus_SmartInverter_Hybrid_PSO_English/IEEE 33-Bus Distribution Network/Bus 18 ==
  In1 : Inport
  Out1 : Outport
  wires:
  In1/1 -> Out1/1

== system IEEE33bus_SmartInverter_Hybrid_PSO_English/IEEE 33-Bus Distribution Network/Bus 19 ==
  In1 : Inport
  Out1 : Outport
  wires:
  In1/1 -> Out1/1

== system IEEE33bus_SmartInverter_Hybrid_PSO_English/IEEE 33-Bus Distribution Network/Bus 2 ==
  In1 : Inport
  Out1 : Outport
  wires:
  In1/1 -> Out1/1

== system IEEE33bus_SmartInverter_Hybrid_PSO_English/IEEE 33-Bus Distribution Network/Bus 20 ==
  In1 : Inport
  Out1 : Outport
  wires:
  In1/1 -> Out1/1

== system IEEE33bus_SmartInverter_Hybrid_PSO_English/IEEE 33-Bus Distribution Network/Bus 21 ==
  In1 : Inport
  Out1 : Outport
  wires:
  In1/1 -> Out1/1

== system IEEE33bus_SmartInverter_Hybrid_PSO_English/IEEE 33-Bus Distribution Network/Bus 22 ==
  In1 : Inport
  Out1 : Outport
  wires:
  In1/1 -> Out1/1

== system IEEE33bus_SmartInverter_Hybrid_PSO_English/IEEE 33-Bus Distribution Network/Bus 23 ==
  In1 : Inport
  Out1 : Outport
  wires:
  In1/1 -> Out1/1

== system IEEE33bus_SmartInverter_Hybrid_PSO_English/IEEE 33-Bus Distribution Network/Bus 24 ==
  In1 : Inport
  Out1 : Outport
  wires:
  In1/1 -> Out1/1

== system IEEE33bus_SmartInverter_Hybrid_PSO_English/IEEE 33-Bus Distribution Network/Bus 25 ==
  In1 : Inport
  Out1 : Outport
  wires:
  In1/1 -> Out1/1

== system IEEE33bus_SmartInverter_Hybrid_PSO_English/IEEE 33-Bus Distribution Network/Bus 26 ==
  In1 : Inport
  Out1 : Outport
  wires:
  In1/1 -> Out1/1

== system IEEE33bus_SmartInverter_Hybrid_PSO_English/IEEE 33-Bus Distribution Network/Bus 27 ==
  In1 : Inport
  Out1 : Outport
  wires:
  In1/1 -> Out1/1

== system IEEE33bus_SmartInverter_Hybrid_PSO_English/IEEE 33-Bus Distribution Network/Bus 28 ==
  In1 : Inport
  Out1 : Outport
  wires:
  In1/1 -> Out1/1

== system IEEE33bus_SmartInverter_Hybrid_PSO_English/IEEE 33-Bus Distribution Network/Bus 29 ==
  In1 : Inport
  Out1 : Outport
  wires:
  In1/1 -> Out1/1

== system IEEE33bus_SmartInverter_Hybrid_PSO_English/IEEE 33-Bus Distribution Network/Bus 3 ==
  In1 : Inport
  Out1 : Outport
  wires:
  In1/1 -> Out1/1

== system IEEE33bus_SmartInverter_Hybrid_PSO_English/IEEE 33-Bus Distribution Network/Bus 30 ==
  In1 : Inport
  Out1 : Outport
  wires:
  In1/1 -> Out1/1

== system IEEE33bus_SmartInverter_Hybrid_PSO_English/IEEE 33-Bus Distribution Network/Bus 31 ==
  In1 : Inport
  Out1 : Outport
  wires:
  In1/1 -> Out1/1

== system IEEE33bus_SmartInverter_Hybrid_PSO_English/IEEE 33-Bus Distribution Network/Bus 32 ==
  In1 : Inport
  Out1 : Outport
  wires:
  In1/1 -> Out1/1

== system IEEE33bus_SmartInverter_Hybrid_PSO_English/IEEE 33-Bus Distribution Network/Bus 33 ==
  In1 : Inport
  Out1 : Outport
  wires:
  In1/1 -> Out1/1

== system IEEE33bus_SmartInverter_Hybrid_PSO_English/IEEE 33-Bus Distribution Network/Bus 4 ==
  In1 : Inport
  Out1 : Outport
  wires:
  In1/1 -> Out1/1

== system IEEE33bus_SmartInverter_Hybrid_PSO_English/IEEE 33-Bus Distribution Network/Bus 5 ==
  In1 : Inport
  Out1 : Outport
  wires:
  In1/1 -> Out1/1

== system IEEE33bus_SmartInverter_Hybrid_PSO_English/IEEE 33-Bus Distribution Network/Bus 6 ==
  In1 : Inport
  Out1 : Outport
  wires:
  In1/1 -> Out1/1

== system IEEE33bus_SmartInverter_Hybrid_PSO_English/IEEE 33-Bus Distribution Network/Bus 7 ==
  In1 : Inport
  Out1 : Outport
  wires:
  In1/1 -> Out1/1

== system IEEE33bus_SmartInverter_Hybrid_PSO_English/IEEE 33-Bus Distribution Network/Bus 8 ==
  In1 : Inport
  Out1 : Outport
  wires:
  In1/1 -> Out1/1

== system IEEE33bus_SmartInverter_Hybrid_PSO_English/IEEE 33-Bus Distribution Network/Bus 9 ==
  In1 : Inport
  Out1 : Outport
  wires:
  In1/1 -> Out1/1

== system IEEE33bus_SmartInverter_Hybrid_PSO_English/IEEE 33-Bus Distribution Network/Load at Bus 18 ==
  In1 : Inport
  Out1 : Outport
  wires:
  In1/1 -> Out1/1

== system IEEE33bus_SmartInverter_Hybrid_PSO_English/IEEE 33-Bus Distribution Network/Load at Bus 22 ==
  In1 : Inport
  Out1 : Outport
  wires:
  In1/1 -> Out1/1

== system IEEE33bus_SmartInverter_Hybrid_PSO_English/IEEE 33-Bus Distribution Network/Load at Bus 25 ==
  In1 : Inport
  Out1 : Outport
  wires:
  In1/1 -> Out1/1

== system IEEE33bus_SmartInverter_Hybrid_PSO_English/IEEE 33-Bus Distribution Network/Load at Bus 33 ==
  In1 : Inport
  Out1 : Outport
  wires:
  In1/1 -> Out1/1

== system IEEE33bus_SmartInverter_Hybrid_PSO_English/IEEE 33-Bus Distribution Network/Three-Phase V-I Measurement ==
  In1 : Inport
  Out1 : Outport
  wires:
  In1/1 -> Out1/1

== system IEEE33bus_SmartInverter_Hybrid_PSO_English/Measurements and Outputs/Active Power ==
  In1 : Inport
  Out1 : Outport
  wires:
  In1/1 -> Out1/1

== system IEEE33bus_SmartInverter_Hybrid_PSO_English/Measurements and Outputs/Bus Currents ==
  In1 : Inport
  Out1 : Outport
  wires:
  In1/1 -> Out1/1

== system IEEE33bus_SmartInverter_Hybrid_PSO_English/Measurements and Outputs/Bus Voltages ==
  In1 : Inport
  Out1 : Outport
  wires:
  In1/1 -> Out1/1

== system IEEE33bus_SmartInverter_Hybrid_PSO_English/Measurements and Outputs/Controller Activation Flags ==
  In1 : Inport
  Out1 : Outport
  wires:
  In1/1 -> Out1/1

== system IEEE33bus_SmartInverter_Hybrid_PSO_English/Measurements and Outputs/PV Curtailment ==
  In1 : Inport
  Out1 : Outport
  wires:
  In1/1 -> Out1/1

== system IEEE33bus_SmartInverter_Hybrid_PSO_English/Measurements and Outputs/Power Losses ==
  In1 : Inport
  Out1 : Outport
  wires:
  In1/1 -> Out1/1

== system IEEE33bus_SmartInverter_Hybrid_PSO_English/Measurements and Outputs/Reactive Power ==
  In1 : Inport
  Out1 : Outport
  wires:
  In1/1 -> Out1/1

== system IEEE33bus_SmartInverter_Hybrid_PSO_English/PV Generation at Selected Buses/MPPT DC-DC Bus 14 ==
  In1 : Inport
  Out1 : Outport
  wires:
  In1/1 -> Out1/1

== system IEEE33bus_SmartInverter_Hybrid_PSO_English/PV Generation at Selected Buses/MPPT DC-DC Bus 18 ==
  In1 : Inport
  Out1 : Outport
  wires:
  In1/1 -> Out1/1

== system IEEE33bus_SmartInverter_Hybrid_PSO_English/PV Generation at Selected Buses/MPPT DC-DC Bus 25 ==
  In1 : Inport
  Out1 : Outport
  wires:
  In1/1 -> Out1/1

== system IEEE33bus_SmartInverter_Hybrid_PSO_English/PV Generation at Selected Buses/MPPT DC-DC Bus 30 ==
  In1 : Inport
  Out1 : Outport
  wires:
  In1/1 -> Out1/1

== system IEEE33bus_SmartInverter_Hybrid_PSO_English/PV Generation at Selected Buses/MPPT DC-DC Bus 33 ==
  In1 : Inport
  Out1 : Outport
  wires:
  In1/1 -> Out1/1

== system IEEE33bus_SmartInverter_Hybrid_PSO_English/PV Generation at Selected Buses/MPPT DC-DC Bus 6 ==
  In1 : Inport
  Out1 : Outport
  wires:
  In1/1 -> Out1/1

== system IEEE33bus_SmartInverter_Hybrid_PSO_English/PV Generation at Selected Buses/PV Array Bus 14 ==
  In1 : Inport
  Out1 : Outport
  wires:
  In1/1 -> Out1/1

== system IEEE33bus_SmartInverter_Hybrid_PSO_English/PV Generation at Selected Buses/PV Array Bus 18 ==
  In1 : Inport
  Out1 : Outport
  wires:
  In1/1 -> Out1/1

== system IEEE33bus_SmartInverter_Hybrid_PSO_English/PV Generation at Selected Buses/PV Array Bus 25 ==
  In1 : Inport
  Out1 : Outport
  wires:
  In1/1 -> Out1/1

== system IEEE33bus_SmartInverter_Hybrid_PSO_English/PV Generation at Selected Buses/PV Array Bus 30 ==
  In1 : Inport
  Out1 : Outport
  wires:
  In1/1 -> Out1/1

== system IEEE33bus_SmartInverter_Hybrid_PSO_English/PV Generation at Selected Buses/PV Array Bus 33 ==
  In1 : Inport
  Out1 : Outport
  wires:
  In1/1 -> Out1/1

== system IEEE33bus_SmartInverter_Hybrid_PSO_English/PV Generation at Selected Buses/PV Array Bus 6 ==
  In1 : Inport
  Out1 : Outport
  wires:
  In1/1 -> Out1/1

== system IEEE33bus_SmartInverter_Hybrid_PSO_English/Performance Indices/Calculate Metrics ==
  In1 : Inport
  Out1 : Outport
  wires:
  In1/1 -> Out1/1

== system IEEE33bus_SmartInverter_Hybrid_PSO_English/Performance Indices/Hosting Capacity ==
  In1 : Inport
  Out1 : Outport
  wires:
  In1/1 -> Out1/1

== system IEEE33bus_SmartInverter_Hybrid_PSO_English/Performance Indices/Max Voltage ==
  In1 : Inport
  Out1 : Outport
  wires:
  In1/1 -> Out1/1

== system IEEE33bus_SmartInverter_Hybrid_PSO_English/Performance Indices/Maximum Voltage Deviation ==
  In1 : Inport
  Out1 : Outport
  wires:
  In1/1 -> Out1/1

== system IEEE33bus_SmartInverter_Hybrid_PSO_English/Performance Indices/Mean Voltage Deviation ==
  In1 : Inport
  Out1 : Outport
  wires:
  In1/1 -> Out1/1

== system IEEE33bus_SmartInverter_Hybrid_PSO_English/Performance Indices/Min Voltage ==
  In1 : Inport
  Out1 : Outport
  wires:
  In1/1 -> Out1/1

== system IEEE33bus_SmartInverter_Hybrid_PSO_English/Performance Indices/Number of Voltage Violations ==
  In1 : Inport
  Out1 : Outport
  wires:
  In1/1 -> Out1/1

== system IEEE33bus_SmartInverter_Hybrid_PSO_English/Performance Indices/PSO Objective Function ==
  In1 : Inport
  Out1 : Outport
  wires:
  In1/1 -> Out1/1

== system IEEE33bus_SmartInverter_Hybrid_PSO_English/Performance Indices/PV Curtailment ==
  In1 : Inport
  Out1 : Outport
  wires:
  In1/1 -> Out1/1

== system IEEE33bus_SmartInverter_Hybrid_PSO_English/Performance Indices/Quasi-static Voltage Recovery Steps ==
  In1 : Inport
  Out1 : Outport
  wires:
  In1/1 -> Out1/1

== system IEEE33bus_SmartInverter_Hybrid_PSO_English/Performance Indices/Save Tables and Figures ==
  In1 : Inport
  Out1 : Outport
  wires:
  In1/1 -> Out1/1

== system IEEE33bus_SmartInverter_Hybrid_PSO_English/Performance Indices/Total Power Loss ==
  In1 : Inport
  Out1 : Outport
  wires:
  In1/1 -> Out1/1

== system IEEE33bus_SmartInverter_Hybrid_PSO_English/Results and Analysis/Final Result Dashboard ==
  In1 : Inport
  Out1 : Outport
  wires:
  In1/1 -> Out1/1

== system IEEE33bus_SmartInverter_Hybrid_PSO_English/Results and Analysis/PSO Convergence Plot ==
  In1 : Inport
  Out1 : Outport
  wires:
  In1/1 -> Out1/1

== system IEEE33bus_SmartInverter_Hybrid_PSO_English/Results and Analysis/PV Curtailment Comparison ==
  In1 : Inport
  Out1 : Outport
  wires:
  In1/1 -> Out1/1

== system IEEE33bus_SmartInverter_Hybrid_PSO_English/Results and Analysis/PV Hosting Capacity ==
  In1 : Inport
  Out1 : Outport
  wires:
  In1/1 -> Out1/1

== system IEEE33bus_SmartInverter_Hybrid_PSO_English/Results and Analysis/Power Loss Comparison ==
  In1 : Inport
  Out1 : Outport
  wires:
  In1/1 -> Out1/1

== system IEEE33bus_SmartInverter_Hybrid_PSO_English/Results and Analysis/Voltage Profile Plot ==
  In1 : Inport
  Out1 : Outport
  wires:
  In1/1 -> Out1/1

== system IEEE33bus_SmartInverter_Hybrid_PSO_English/Results and Analysis/Voltage Violation Count ==
  In1 : Inport
  Out1 : Outport
  wires:
  In1/1 -> Out1/1

== system IEEE33bus_SmartInverter_Hybrid_PSO_English/Simulation Scenarios/Control Modes ==
  In1 : Inport
  Out1 : Outport
  wires:
  In1/1 -> Out1/1

== system IEEE33bus_SmartInverter_Hybrid_PSO_English/Simulation Scenarios/Irradiance and Load Conditions ==
  In1 : Inport
  Out1 : Outport
  wires:
  In1/1 -> Out1/1

== system IEEE33bus_SmartInverter_Hybrid_PSO_English/Simulation Scenarios/PV Penetration Levels ==
  In1 : Inport
  Out1 : Outport
  wires:
  In1/1 -> Out1/1

== system IEEE33bus_SmartInverter_Hybrid_PSO_English/Smart Inverter - VSI/DC Link ==
  In1 : Inport
  Out1 : Outport
  wires:
  In1/1 -> Out1/1

== system IEEE33bus_SmartInverter_Hybrid_PSO_English/Smart Inverter - VSI/Grid Synchronization PLL ==
  In1 : Inport
  Out1 : Outport
  wires:
  In1/1 -> Out1/1

== system IEEE33bus_SmartInverter_Hybrid_PSO_English/Smart Inverter - VSI/Inverter Capability Limit ==
  In1 : Inport
  Out1 : Outport
  wires:
  In1/1 -> Out1/1

== system IEEE33bus_SmartInverter_Hybrid_PSO_English/Smart Inverter - VSI/LCL Filter ==
  In1 : Inport
  Out1 : Outport
  wires:
  In1/1 -> Out1/1

== system IEEE33bus_SmartInverter_Hybrid_PSO_English/Smart Inverter - VSI/P-Q Reference Input ==
  In1 : Inport
  Out1 : Outport
  wires:
  In1/1 -> Out1/1

== system IEEE33bus_SmartInverter_Hybrid_PSO_English/Smart Inverter - VSI/Three-Phase VSI ==
  In1 : Inport
  Out1 : Outport
  wires:
  In1/1 -> Out1/1
